simulink model "BCMotor"  (R2021a)
settings: Solver=ode23  StartTime=0  StopTime=0.6  RelTol=1e-5
values from neighbouring files (symbols this model uses):
  Ce = 0.96    [BCMotor_params.mat]    (also in p_3_6.m = 0.058; paragraph 3_3_1.mat = 0.153; paragraph 3_3_2.mat = 0.153; paragraph 3_3_3.mat = 0.153)
  Cm = 1.85    [BCMotor_params.mat]    (also in p_3_6.m = 0.057; paragraph 3_3_1.mat = 0.156; paragraph 3_3_2.mat = 0.156; paragraph 3_3_3.mat = 0.156)
  J = 2.02e-05    [BCMotor_params.mat]    (also in p_3_6.m = 8.4e-05; paragraph 3_3_1.mat = 0.000122; paragraph 3_3_2.mat = 0.000122; paragraph 3_3_3.mat = 0.000122)
  L = 0.187    [BCMotor_params.mat]
  P = 8    [BCMotor_params.mat]
  R = 0.45    [BCMotor_params.mat]    (also in p_3_6.m = TuningGoal.StepResp('SpeedRef', 'Speed', 0.2, 0); robustPidController.m = TuningGoal.StepResp('SpeedRef', 'Speed', 0.2, 0); robustPidControllerForAngle.m = TuningGoal.StepResp('AngleRef', 'Angle', 0.2, 0))
undefined symbols (not defined in the file or in its folder): kd, ki, kp
libraries: checkpacklib x2, pid_lib x2
settings Model: Creator=slagt  LastModifiedBy=slagt
settings DataIOCC: SaveFormat=StructureWithTime
settings OptimizationCC: BlockReduction=off  BufferReuse=off
settings DebuggingCC: AlgebraicLoopMsg=none  UnconnectedInputMsg=none  UnconnectedOutputMsg=none  UnconnectedLineMsg=none

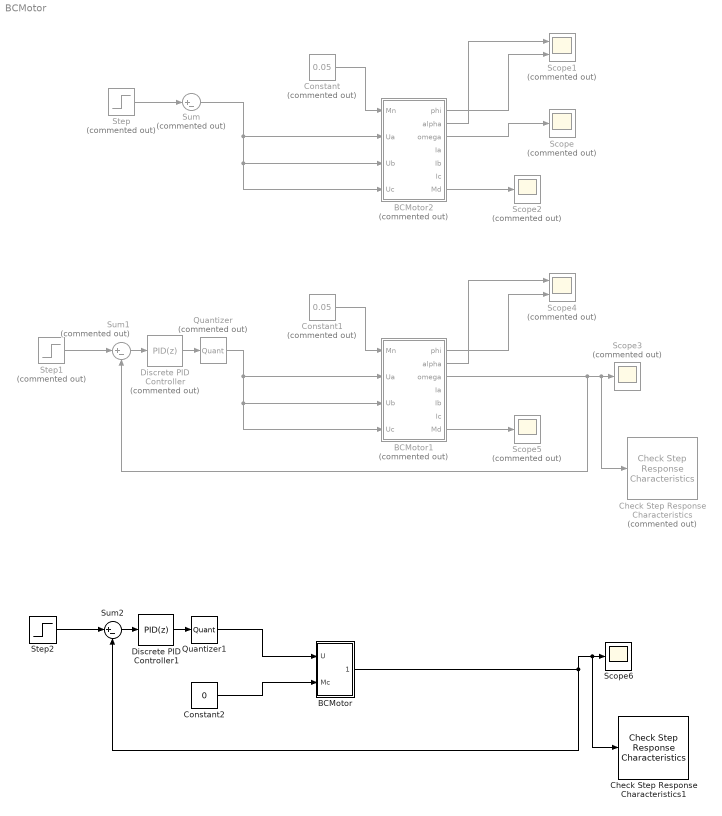
== system BCMotor ==
  BCMotor : Subsystem
  BCMotor1 : Subsystem  Commented=on
  BCMotor2 : Subsystem  Commented=on
  Check Step Response Characteristics : checkpacklib/Check Step Response  Characteristics  Commented=on  InstantiateOnLoad=on  enabled=on  stopWhenAssertionFail=off  export=off  ViewDlgPos=[]  OpenViewOnLoad=off  LaunchViewOnOpen=off  TimeUnits=seconds  EnableStepResponseBound=on  InitialValue=0  FinalValue=1  StepTime=0  RiseTime=0.2  PercentRise=80  SettlingTime=0.4  PercentSettling=1  PercentOvershoot=10  PercentUndershoot=1
      settings: SourceProductBaseCode=CT,ID,MT,SO
  Check Step Response Characteristics1 : checkpacklib/Check Step Response  Characteristics  InstantiateOnLoad=on  enabled=on  stopWhenAssertionFail=off  export=off  ViewDlgPos=[]  OpenViewOnLoad=off  LaunchViewOnOpen=off  TimeUnits=seconds  EnableStepResponseBound=on  InitialValue=0  FinalValue=1  StepTime=0  RiseTime=0.2  PercentRise=80  SettlingTime=0.4  PercentSettling=1  PercentOvershoot=10  PercentUndershoot=1
      settings: SourceProductBaseCode=CT,ID,MT,SO
  Constant : Constant  Commented=on  Value=0.05
  Constant1 : Constant  Commented=on  Value=0.05
  Constant2 : Constant  Value=0
  Discrete PID Controller : pid_lib/PID Controller  Commented=on  Controller=PID  Form=Parallel  TimeDomain=Discrete-time  UseExternalTs=off  SampleTime=10^-5  IntegratorMethod=Forward Euler  FilterMethod=Forward Euler  ControllerParametersSource=internal  P=kp  I=ki  D=kd  UseFilter=on  N=100  TunerSelectOption=Transfer Function Based (PID Tuner App)  InitialConditionSource=internal  InitialConditionForIntegrator=0  InitialConditionForFilter=0  DifferentiatorICPrevScaledInput=0  ExternalReset=none  TrackingMode=off  Kt=1  LimitOutput=off  SatLimitsSource=internal  UpperSaturationLimit=inf  LowerSaturationLimit=-inf  LinearizeAsGain=off  AntiWindupMode=none  Kb=1  POutMin=[]  POutMax=[]  IOutMin=[]  IOutMax=[]  DOutMin=[]  DOutMax=[]  NOutMin=[]  NOutMax=[]  SumOutMin=[]  SumOutMax=[]  SaturationOutMin=[]  SaturationOutMax=[]  PParamMin=[]  PParamMax=[]  IParamMin=[]  IParamMax=[]  DParamMin=[]  DParamMax=[]  NParamMin=[]  NParamMax=[]  KbParamMin=[]  KbParamMax=[]  KtParamMin=[]  KtParamMax=[]  KbOutMin=[]  KbOutMax=[]  KtOutMin=[]  KtOutMax=[]  IntegratorOutMin=[]  IntegratorOutMax=[]  FilterOutMin=[]  FilterOutMax=[]  SumI1OutMin=[]  SumI1OutMax=[]  SumI2OutMin=[]  SumI2OutMax=[]  SumI3OutMin=[]  SumI3OutMax=[]  SumI4OutMin=[]  SumI4OutMax=[]  SumDOutMin=[]  SumDOutMax=[]  DifferentiatorOutMin=[]  DifferentiatorOutMax=[]  FilterDiffOutCoefMin=[]  FilterDiffOutCoefMax=[]  ReciprocalOutMin=[]  ReciprocalOutMax=[]  SumDenOutMin=[]  SumDenOutMax=[]  SumNumOutMin=[]  SumNumOutMax=[]  DivideOutMin=[]  DivideOutMax=[]  UdiffTsProdOutMin=[]  UdiffTsProdOutMax=[]  NTsProdOutMin=[]  NTsProdOutMax=[]  UintegralTsProdOutMin=[]  UintegralTsProdOutMax=[]  UngainTsProdOutMin=[]  UngainTsProdOutMax=[]  IntegratorContinuousStateAttributes=''  IntegratorStateMustResolveToSignalObject=off  IntegratorRTWStateStorageClass=Auto  FilterContinuousStateAttributes=''  FilterStateMustResolveToSignalObject=off  FilterRTWStateStorageClass=Auto  ParallelPVariant=InternalParameters  IdealPVariant=Disabled  IVariant=InternalParameters  DVariant=InternalParameters  IntegratorVariant=Discrete  SatVariant=Disabled  AWVariant=Passthrough  PCopyVariant=Disabled  TRVariant=Disabled  FdbkBlocksVariant=Forward  IdealPFdbkVariant=Disabled  SatFdbkVariant=Disabled  DerivativeFilterVariant=ForwardEulerFilter  NVariant=InternalParameters  NCopyVariant=Disabled  FilterICVariant=InternalICsFilter  IntegratorICVariant=InternalICs  ExternalResetVariant=Disabled  TRSumVariant=Passthrough  SumFdbkVariant=Disabled  SumVariant=Sum_PID  TsampFilterVariant=InternalTs  TsampNgainVariant=Passthrough  TsampIntegralVariant=Passthrough  ExternalSaturationOutDataTypeStr=Inherit: Same as second input
  Discrete PID Controller1 : pid_lib/PID Controller  Controller=PID  Form=Parallel  TimeDomain=Discrete-time  UseExternalTs=off  SampleTime=10^-6  IntegratorMethod=Forward Euler  FilterMethod=Forward Euler  ControllerParametersSource=internal  P=kp  I=ki  D=kd  UseFilter=on  N=100  TunerSelectOption=Transfer Function Based (PID Tuner App)  InitialConditionSource=internal  InitialConditionForIntegrator=0  InitialConditionForFilter=0  DifferentiatorICPrevScaledInput=0  ExternalReset=none  TrackingMode=off  Kt=1  LimitOutput=off  SatLimitsSource=internal  UpperSaturationLimit=inf  LowerSaturationLimit=-inf  LinearizeAsGain=off  AntiWindupMode=none  Kb=1  POutMin=[]  POutMax=[]  IOutMin=[]  IOutMax=[]  DOutMin=[]  DOutMax=[]  NOutMin=[]  NOutMax=[]  SumOutMin=[]  SumOutMax=[]  SaturationOutMin=[]  SaturationOutMax=[]  PParamMin=[]  PParamMax=[]  IParamMin=[]  IParamMax=[]  DParamMin=[]  DParamMax=[]  NParamMin=[]  NParamMax=[]  KbParamMin=[]  KbParamMax=[]  KtParamMin=[]  KtParamMax=[]  KbOutMin=[]  KbOutMax=[]  KtOutMin=[]  KtOutMax=[]  IntegratorOutMin=[]  IntegratorOutMax=[]  FilterOutMin=[]  FilterOutMax=[]  SumI1OutMin=[]  SumI1OutMax=[]  SumI2OutMin=[]  SumI2OutMax=[]  SumI3OutMin=[]  SumI3OutMax=[]  SumI4OutMin=[]  SumI4OutMax=[]  SumDOutMin=[]  SumDOutMax=[]  DifferentiatorOutMin=[]  DifferentiatorOutMax=[]  FilterDiffOutCoefMin=[]  FilterDiffOutCoefMax=[]  ReciprocalOutMin=[]  ReciprocalOutMax=[]  SumDenOutMin=[]  SumDenOutMax=[]  SumNumOutMin=[]  SumNumOutMax=[]  DivideOutMin=[]  DivideOutMax=[]  UdiffTsProdOutMin=[]  UdiffTsProdOutMax=[]  NTsProdOutMin=[]  NTsProdOutMax=[]  UintegralTsProdOutMin=[]  UintegralTsProdOutMax=[]  UngainTsProdOutMin=[]  UngainTsProdOutMax=[]  IntegratorContinuousStateAttributes=''  IntegratorStateMustResolveToSignalObject=off  IntegratorRTWStateStorageClass=Auto  FilterContinuousStateAttributes=''  FilterStateMustResolveToSignalObject=off  FilterRTWStateStorageClass=Auto  ParallelPVariant=InternalParameters  IdealPVariant=Disabled  IVariant=InternalParameters  DVariant=InternalParameters  IntegratorVariant=Discrete  SatVariant=Disabled  AWVariant=Passthrough  PCopyVariant=Disabled  TRVariant=Disabled  FdbkBlocksVariant=Forward  IdealPFdbkVariant=Disabled  SatFdbkVariant=Disabled  DerivativeFilterVariant=ForwardEulerFilter  NVariant=InternalParameters  NCopyVariant=Disabled  FilterICVariant=InternalICsFilter  IntegratorICVariant=InternalICs  ExternalResetVariant=Disabled  TRSumVariant=Passthrough  SumFdbkVariant=Disabled  SumVariant=Sum_PID  TsampFilterVariant=InternalTs  TsampNgainVariant=Passthrough  TsampIntegralVariant=Passthrough  ExternalSaturationOutDataTypeStr=Inherit: Same as second input
  Quantizer : Quantizer  Commented=on  QuantizationInterval=0.02  LinearizeAsGain=off
  Quantizer1 : Quantizer  QuantizationInterval=0.001  LinearizeAsGain=off
  Scope{,2..3,5} (4 alike) : Scope  Commented=on
  Scope1 : Scope  Commented=on  NumInputPorts=2
  Scope4 : Scope  Commented=on  NumInputPorts=2
  Scope6 : Scope
  Step : Step  Commented=on  Time=0  After=24  SampleTime=0
  Step1 : Step  Commented=on  Time=0  After=24  SampleTime=0
  Step2 : Step  Time=0  SampleTime=0
  Sum : Sum  Commented=on  Inputs=|+-
  Sum1 : Sum  Commented=on  Inputs=|+-
  Sum2 : Sum  Inputs=|+-
  wires:
  Step/1 -> Sum/1
  Sum/1 -> BCMotor2/2(Ua), BCMotor2/3(Ub), BCMotor2/4(Uc)
  BCMotor2/3(omega) -> Scope/1
  Constant/1 -> BCMotor2/1(Mn)
  BCMotor2/2(alpha) -> Scope1/1
  BCMotor2/1(phi) -> Scope1/2
  BCMotor2/7(Md) -> Scope2/1
  BCMotor1/2(alpha) -> Scope4/1
  BCMotor1/7(Md) -> Scope5/1
  Step1/1 -> Sum1/1
  Constant1/1 -> BCMotor1/1(Mn)
  Sum1/1 -> Discrete PID Controller/1
  BCMotor1/1(phi) -> Scope4/2
  Discrete PID Controller/1 -> Quantizer/1
  BCMotor1/3(omega) -> Sum1/2, Check Step Response Characteristics/1, Scope3/1
  Quantizer/1 -> BCMotor1/2(Ua), BCMotor1/3(Ub), BCMotor1/4(Uc)
  Step2/1 -> Sum2/1
  Discrete PID Controller1/1 -> Quantizer1/1
  Sum2/1 -> Discrete PID Controller1/1
  BCMotor/1(omega) -> Check Step Response Characteristics1/1, Scope6/1, Sum2/2
  Quantizer1/1 -> BCMotor/1(U)
  Constant2/1 -> BCMotor/2(Mc)

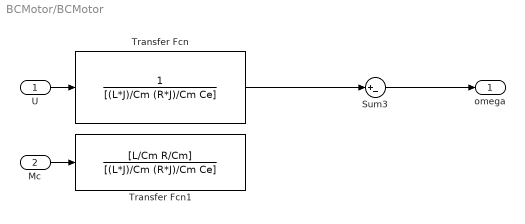
== system BCMotor/BCMotor ==
  U : Inport
  Mc : Inport  Port=2
  Sum3 : Sum  Inputs=|+-
  Transfer Fcn : TransferFcn  Denominator=[(L*J)/Cm (R*J)/Cm Ce]
  Transfer Fcn1 : TransferFcn  Numerator=[L/Cm R/Cm]  Denominator=[(L*J)/Cm (R*J)/Cm Ce]
  omega : Outport
  wires:
  Mc/1 -> Transfer Fcn1/1
  Sum3/1 -> omega/1
  Transfer Fcn/1 -> Sum3/1
  U/1 -> Transfer Fcn/1

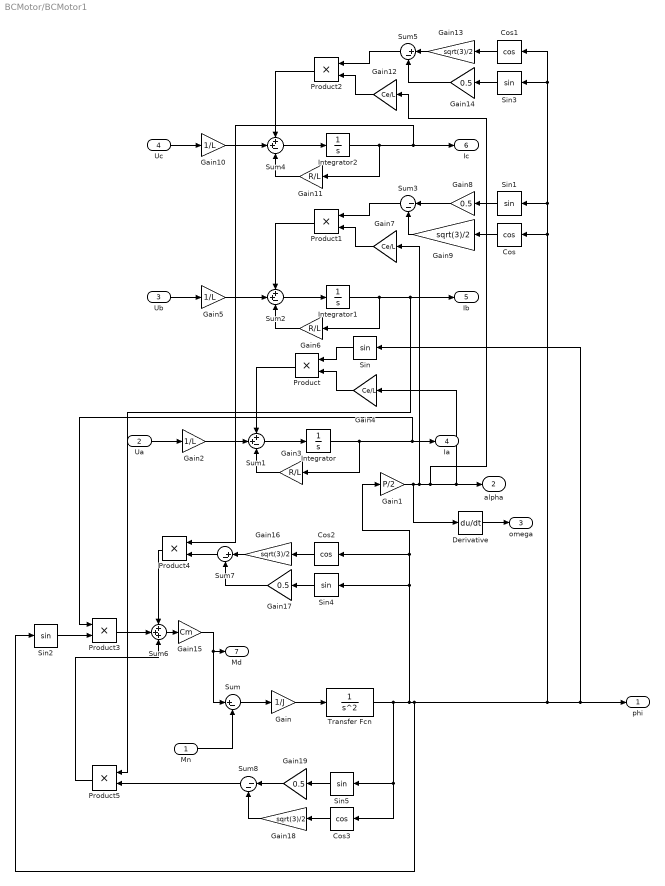
== system BCMotor/BCMotor1 ==
  Mn : Inport
  Ua : Inport  Port=2
  Ub : Inport  Port=3
  Uc : Inport  Port=4
  Cos{,1..3} (4 alike) : Trigonometry  Operator=cos
  Derivative : Derivative
  Gain : Gain  Gain=1/J
  Gain1 : Gain  Gain=P/2
  Gain10 : Gain  Gain=1/L
  Gain11 : Gain  Gain=R/L
  Gain12 : Gain  Gain=Ce/L
  Gain{9,13,16,18} (4 alike) : Gain  Gain=sqrt(3)/2
  Gain{8,14,17,19} (4 alike) : Gain  Gain=0.5
  Gain15 : Gain  Gain=Cm
  Gain2 : Gain  Gain=1/L
  Gain3 : Gain  Gain=R/L
  Gain4 : Gain  Gain=Ce/L
  Gain5 : Gain  Gain=1/L
  Gain6 : Gain  Gain=R/L
  Gain7 : Gain  Gain=Ce/L
  Integrator : Integrator
  Integrator1 : Integrator
  Integrator2 : Integrator
  Product{,1..5} (6 alike) : Product
  Sin{,1..5} (6 alike) : Trigonometry
  Sum : Sum  Inputs=|+-
  Sum1 : Sum  Inputs=++-
  Sum2 : Sum  Inputs=++-
  Sum3 : Sum  Inputs=|--
  Sum4 : Sum  Inputs=++-
  Sum5 : Sum  Inputs=|+-
  Sum6 : Sum  Inputs=+++
  Sum7 : Sum  Inputs=|+-
  Sum8 : Sum  Inputs=|--
  Transfer Fcn : TransferFcn  Denominator=[1 0 0]
  phi : Outport
  alpha : Outport  Port=2
  omega : Outport  Port=3
  Ia : Outport  Port=4
  Ib : Outport  Port=5
  Ic : Outport  Port=6
  Md : Outport  Port=7
  wires:
  Cos3/1 -> Gain18/1
  Integrator/1 -> Gain3/1, Ia/1, Product3/1
  Product2/1 -> Sum4/1
  Mn/1 -> Sum/2
  Sin4/1 -> Gain17/1
  Sin5/1 -> Gain19/1
  Sum6/1 -> Gain15/1
  Sum1/1 -> Integrator/1
  Integrator1/1 -> Gain6/1, Ib/1, Product5/1
  Gain16/1 -> Sum7/1
  Ub/1 -> Gain5/1
  Sum3/1 -> Product1/1
  Gain11/1 -> Sum4/3
  Gain17/1 -> Sum7/2
  Gain2/1 -> Sum1/2
  Gain13/1 -> Sum5/1
  Ua/1 -> Gain2/1
  Sin/1 -> Product/1
  Sum/1 -> Gain/1
  Product/1 -> Sum1/1
  Gain18/1 -> Sum8/2
  Gain3/1 -> Sum1/3
  Gain4/1 -> Product/2
  Product5/1 -> Sum6/3
  Sin3/1 -> Gain14/1
  Sum8/1 -> Product5/2
  Gain10/1 -> Sum4/2
  Sin2/1 -> Product3/2
  Gain12/1 -> Product2/2
  Sum7/1 -> Product4/2
  Gain6/1 -> Sum2/3
  Gain/1 -> Transfer Fcn/1
  Cos1/1 -> Gain13/1
  Gain8/1 -> Sum3/1
  Gain7/1 -> Product1/2
  Cos/1 -> Gain9/1
  Cos2/1 -> Gain16/1
  Gain5/1 -> Sum2/2
  Product1/1 -> Sum2/1
  Sum2/1 -> Integrator1/1
  Integrator2/1 -> Gain11/1, Ic/1, Product4/1
  Gain19/1 -> Sum8/1
  Product4/1 -> Sum6/1
  Sum4/1 -> Integrator2/1
  Uc/1 -> Gain10/1
  Gain14/1 -> Sum5/2
  Sum5/1 -> Product2/1
  Gain9/1 -> Sum3/2
  Sin1/1 -> Gain8/1
  Product3/1 -> Sum6/2
  Gain15/1 -> Md/1, Sum/1
  Gain1/1 -> Derivative/1, Gain12/1, alpha/1, Gain4/1, Gain7/1
  Derivative/1 -> omega/1
  Transfer Fcn/1 -> Cos3/1, Sin5/1, Gain1/1, Cos2/1, Sin4/1, Sin2/1, Cos1/1, Sin3/1, Sin1/1, Cos/1, Sin/1, phi/1

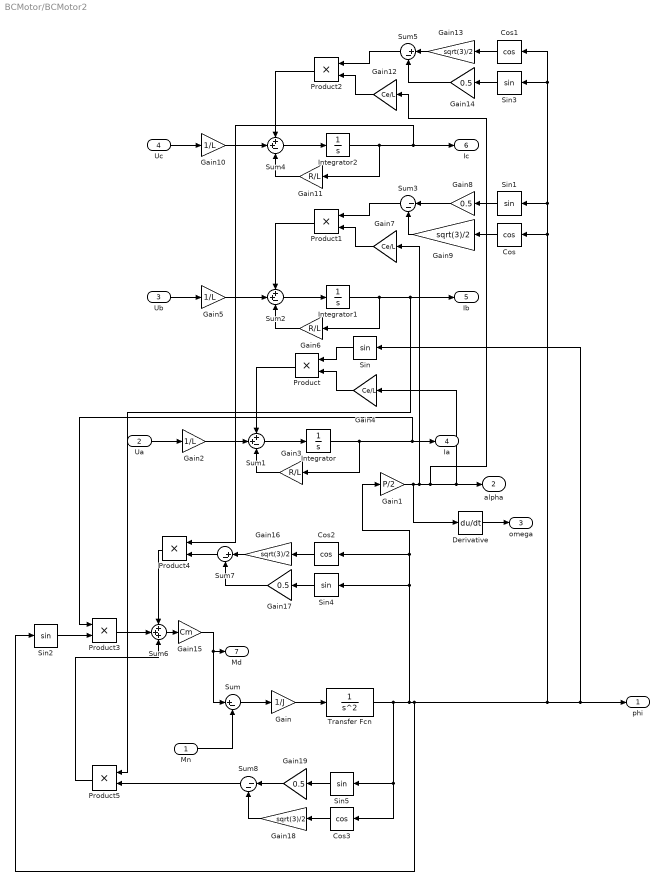
== system BCMotor/BCMotor2 ==
  Mn : Inport
  Ua : Inport  Port=2
  Ub : Inport  Port=3
  Uc : Inport  Port=4
  Cos{,1..3} (4 alike) : Trigonometry  Operator=cos
  Derivative : Derivative
  Gain : Gain  Gain=1/J
  Gain1 : Gain  Gain=P/2
  Gain10 : Gain  Gain=1/L
  Gain11 : Gain  Gain=R/L
  Gain12 : Gain  Gain=Ce/L
  Gain{9,13,16,18} (4 alike) : Gain  Gain=sqrt(3)/2
  Gain{8,14,17,19} (4 alike) : Gain  Gain=0.5
  Gain15 : Gain  Gain=Cm
  Gain2 : Gain  Gain=1/L
  Gain3 : Gain  Gain=R/L
  Gain4 : Gain  Gain=Ce/L
  Gain5 : Gain  Gain=1/L
  Gain6 : Gain  Gain=R/L
  Gain7 : Gain  Gain=Ce/L
  Integrator : Integrator
  Integrator1 : Integrator
  Integrator2 : Integrator
  Product{,1..5} (6 alike) : Product
  Sin{,1..5} (6 alike) : Trigonometry
  Sum : Sum  Inputs=|+-
  Sum1 : Sum  Inputs=++-
  Sum2 : Sum  Inputs=++-
  Sum3 : Sum  Inputs=|--
  Sum4 : Sum  Inputs=++-
  Sum5 : Sum  Inputs=|+-
  Sum6 : Sum  Inputs=+++
  Sum7 : Sum  Inputs=|+-
  Sum8 : Sum  Inputs=|--
  Transfer Fcn : TransferFcn  Denominator=[1 0 0]
  phi : Outport
  alpha : Outport  Port=2
  omega : Outport  Port=3
  Ia : Outport  Port=4
  Ib : Outport  Port=5
  Ic : Outport  Port=6
  Md : Outport  Port=7
  wires:
  Cos3/1 -> Gain18/1
  Integrator/1 -> Gain3/1, Ia/1, Product3/1
  Product2/1 -> Sum4/1
  Mn/1 -> Sum/2
  Sin4/1 -> Gain17/1
  Sin5/1 -> Gain19/1
  Sum6/1 -> Gain15/1
  Sum1/1 -> Integrator/1
  Integrator1/1 -> Gain6/1, Ib/1, Product5/1
  Gain16/1 -> Sum7/1
  Ub/1 -> Gain5/1
  Sum3/1 -> Product1/1
  Gain11/1 -> Sum4/3
  Gain17/1 -> Sum7/2
  Gain2/1 -> Sum1/2
  Gain13/1 -> Sum5/1
  Ua/1 -> Gain2/1
  Sin/1 -> Product/1
  Sum/1 -> Gain/1
  Product/1 -> Sum1/1
  Gain18/1 -> Sum8/2
  Gain3/1 -> Sum1/3
  Gain4/1 -> Product/2
  Product5/1 -> Sum6/3
  Sin3/1 -> Gain14/1
  Sum8/1 -> Product5/2
  Gain10/1 -> Sum4/2
  Sin2/1 -> Product3/2
  Gain12/1 -> Product2/2
  Sum7/1 -> Product4/2
  Gain6/1 -> Sum2/3
  Gain/1 -> Transfer Fcn/1
  Cos1/1 -> Gain13/1
  Gain8/1 -> Sum3/1
  Gain7/1 -> Product1/2
  Cos/1 -> Gain9/1
  Cos2/1 -> Gain16/1
  Gain5/1 -> Sum2/2
  Product1/1 -> Sum2/1
  Sum2/1 -> Integrator1/1
  Integrator2/1 -> Gain11/1, Ic/1, Product4/1
  Gain19/1 -> Sum8/1
  Product4/1 -> Sum6/1
  Sum4/1 -> Integrator2/1
  Uc/1 -> Gain10/1
  Gain14/1 -> Sum5/2
  Sum5/1 -> Product2/1
  Gain9/1 -> Sum3/2
  Sin1/1 -> Gain8/1
  Product3/1 -> Sum6/2
  Gain15/1 -> Md/1, Sum/1
  Gain1/1 -> Derivative/1, Gain12/1, alpha/1, Gain4/1, Gain7/1
  Derivative/1 -> omega/1
  Transfer Fcn/1 -> Cos3/1, Sin5/1, Gain1/1, Cos2/1, Sin4/1, Sin2/1, Cos1/1, Sin3/1, Sin1/1, Cos/1, Sin/1, phi/1
